simulink subsystem "subsystem_hall_effect_encoder"  (R2022a)
settings: Solver=VariableStepAuto  StartTime=0.0  StopTime=10.0  RelTol=1e-3
undefined symbols (not defined in the file): cos_amp, cos_center, sin_amp, sin_center
settings Model: Creator=chris  LastModifiedBy=chris

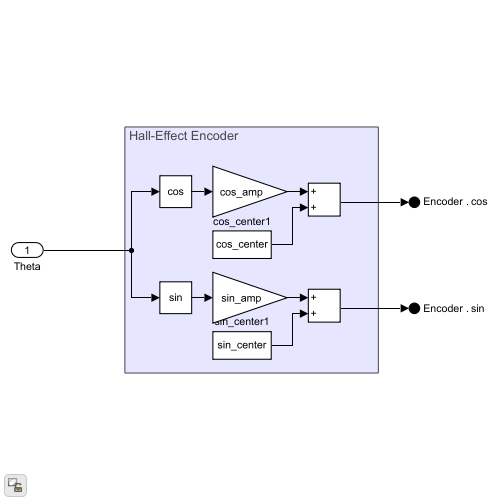
[thumbnail: Simulink's stored preview of the top-level diagram]
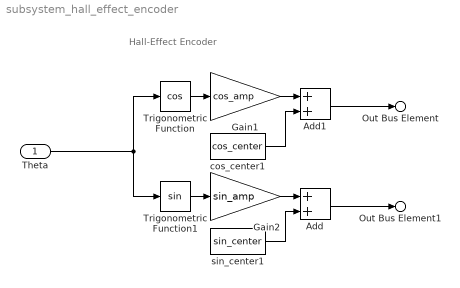
== system subsystem_hall_effect_encoder ==
  note: Hall-Effect Encoder
  Theta : Inport
  Add : Sum
  Add1 : Sum
  Gain1 : Gain  Gain=cos_amp
  Gain2 : Gain  Gain=sin_amp
  Trigonometric Function : Trigonometry  Operator=cos
  Trigonometric Function1 : Trigonometry
  cos_center1 : Constant  Value=cos_center
  sin_center1 : Constant  Value=sin_center
  Out Bus Element : Outport  PortName=Encoder  Element=cos
  Out Bus Element1 : Outport  PortName=Encoder  Element=sin
  wires:
  Trigonometric Function1/1 -> Gain2/1
  Gain1/1 -> Add1/1
  Add1/1 -> Out Bus Element/1
  cos_center1/1 -> Add1/2
  Theta/1 -> Trigonometric Function1/1, Trigonometric Function/1
  Trigonometric Function/1 -> Gain1/1
  sin_center1/1 -> Add/2
  Gain2/1 -> Add/1
  Add/1 -> Out Bus Element1/1
